simulink model "geometric_control_load"  (R2025a)
settings: Solver=ode15s  StartTime=0.0  StopTime=T_total  FixedStep=0.01  RelTol=1e-9
InitFcn:
  | close all;
  | clear all;
  | %% Parameters
  | mQ = 0.5;
  | mL = 0.1;
  | J = [2.32e-3,0,0;0,2.32e-3,0;0,0,4e-3];
  | g = 9.81;
  | e1 = [1;0;0];
  | e2 = [0;1;0];
  | e3 = [0;0;1];
  | l = 1;
  | type_traj = 0; % 0 elliptical, 1 multi-frequency
  | 
  | %% Initial Condition
  | if type_traj == 0
  |     xL = [0;0.8;1];
  |     vL = zeros(3,1);
  |     th = 125*pi/180;
  |     q = [-sin(th);0;cos(th)];
  |     omega = [0;0;0];
  |     R = [1 0 0;0 1 0;0 0 1];
  |     Omega = [0;0;0];
  | else
  |     xL = [0;1;3];
  |     vL = zeros(3,1);
  |     th = 178*pi/180;
  |     q = [-sin(th);0;-cos(th)];
  |     omega = [0;0;0];
  |     R = [-1 0 0;0 1 0;0 0 -1];
  |     Omega = [0;0;0];
  | end
  | 
  | x_0 = [xL; q; reshape(R, 9,1); vL ;omega; Omega];
  | T_total = 10;
settings Model: Creator=fabioruggiero  LastModifiedBy=maist
settings ModelReferenceCC: EnableRefExpFcnMdlSchedulingChecks=on
settings RTWCC: GPUComputeCapability=3.5

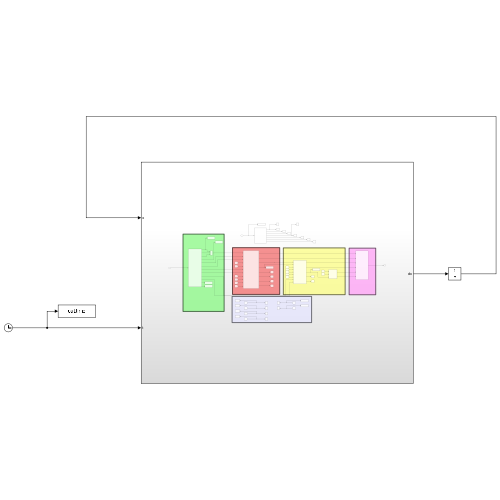
[thumbnail: Simulink's stored preview of the top-level diagram]
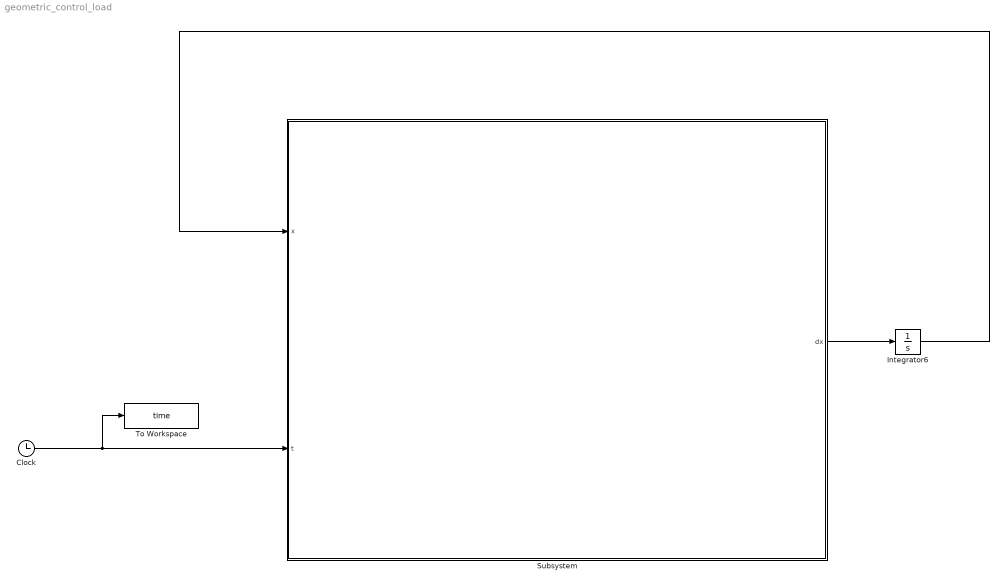
== system geometric_control_load ==
  Clock : Clock
  Integrator6 : Integrator  InitialCondition=x_0
  Subsystem : Subsystem
  To Workspace : ToWorkspace  VariableName=time  SampleTime=-1
      settings: Save2DSignal=2-D array (concatenate along first dimension)
  wires:
  Subsystem/1(dx) -> Integrator6/1
  Integrator6/1 -> Subsystem/1(x)
  Clock/1 -> To Workspace/1, Subsystem/2(t)

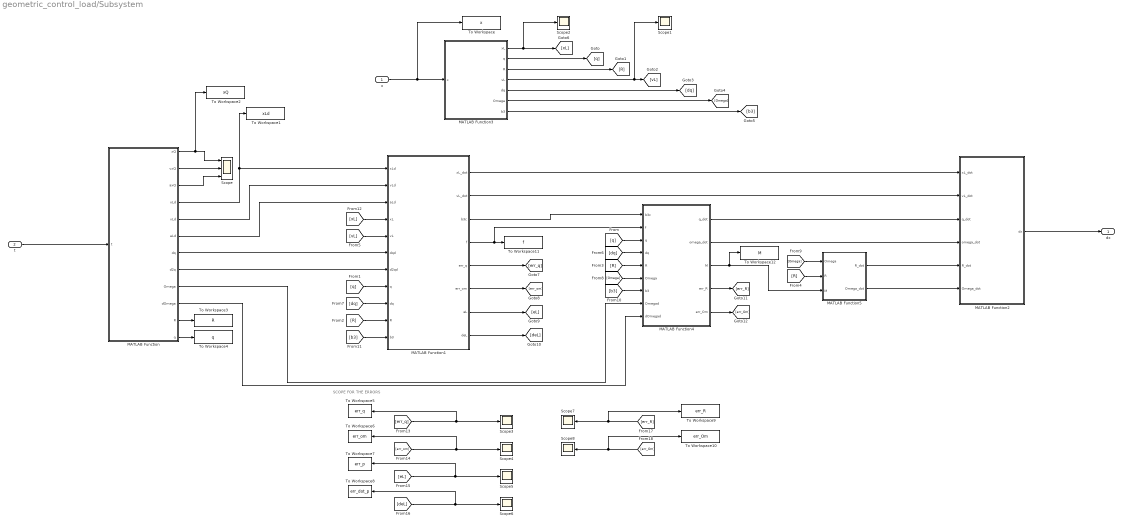
== system geometric_control_load/Subsystem ==
  note: SCOPE FOR THE ERRORS
  x : Inport
  t : Inport  Port=2
  MATLAB Function : MATLAB Function  TreatAsAtomicUnit=on
  MATLAB Function1 : MATLAB Function  TreatAsAtomicUnit=on
  MATLAB Function2 : MATLAB Function  TreatAsAtomicUnit=on
  MATLAB Function3 : MATLAB Function  TreatAsAtomicUnit=on
  MATLAB Function4 : MATLAB Function  TreatAsAtomicUnit=on
  MATLAB Function5 : MATLAB Function  TreatAsAtomicUnit=on
  Scope : Scope  NumInputPorts=3
      settings: ActiveDisplayYMinimum=-2.78929  ActiveDisplayYMaximum=4.74636
  Scope{1..8} (8 alike) : Scope
      Scope1 settings: ActiveDisplayYMinimum=-3.85696  ActiveDisplayYMaximum=4.72111
      Scope2 settings: ActiveDisplayYMinimum=-4.5090813739602247  ActiveDisplayYMaximum=5.0436767590166554
      Scope3 settings: ActiveDisplayYMinimum=-1.0972642217159343  ActiveDisplayYMaximum=1.1831120061993132
      Scope4 settings: ActiveDisplayYMinimum=-1  ActiveDisplayYMaximum=1  DataLoggingVariableName=ScopeData2
      Scope5 settings: ActiveDisplayYMinimum=-6.4063703352333583  ActiveDisplayYMaximum=2.3784855928037065  DataLoggingVariableName=ScopeData3
      Scope6 settings: ActiveDisplayYMinimum=-1  ActiveDisplayYMaximum=1  DataLoggingVariableName=ScopeData4
      Scope7 settings: ActiveDisplayYMinimum=-0.96768549587704089  ActiveDisplayYMaximum=1.1643255351100141  DataLoggingVariableName=ScopeData5
      Scope8 settings: DataLoggingVariableName=ScopeData6
  To Workspace : ToWorkspace  VariableName=x  SampleTime=-1
      settings: Save2DSignal=2-D array (concatenate along first dimension)
  To Workspace1 : ToWorkspace  VariableName=xLd  SampleTime=-1
      settings: Save2DSignal=2-D array (concatenate along first dimension)
  To Workspace10 : ToWorkspace  VariableName=err_Om  SampleTime=-1
      settings: Save2DSignal=2-D array (concatenate along first dimension)
  To Workspace11 : ToWorkspace  VariableName=f  SampleTime=-1
      settings: Save2DSignal=2-D array (concatenate along first dimension)
  To Workspace12 : ToWorkspace  VariableName=M  SampleTime=-1
      settings: Save2DSignal=2-D array (concatenate along first dimension)
  To Workspace2 : ToWorkspace  VariableName=xQ  SampleTime=-1
      settings: Save2DSignal=2-D array (concatenate along first dimension)
  To Workspace3 : ToWorkspace  VariableName=R  SampleTime=-1
  To Workspace4 : ToWorkspace  VariableName=q  SampleTime=-1
      settings: Save2DSignal=2-D array (concatenate along first dimension)
  To Workspace5 : ToWorkspace  VariableName=err_q  SampleTime=-1
      settings: Save2DSignal=2-D array (concatenate along first dimension)
  To Workspace6 : ToWorkspace  VariableName=err_om  SampleTime=-1
      settings: Save2DSignal=2-D array (concatenate along first dimension)
  To Workspace7 : ToWorkspace  VariableName=err_p  SampleTime=-1
      settings: Save2DSignal=2-D array (concatenate along first dimension)
  To Workspace8 : ToWorkspace  VariableName=err_dot_p  SampleTime=-1
      settings: Save2DSignal=2-D array (concatenate along first dimension)
  To Workspace9 : ToWorkspace  VariableName=err_R  SampleTime=-1
      settings: Save2DSignal=2-D array (concatenate along first dimension)
  dx : Outport
  wires:
  MATLAB Function2/1(dx) -> dx/1
  x/1 -> To Workspace/1, MATLAB Function3/1(x)
  MATLAB Function3/5(dq) -> [dq]
  MATLAB Function3/7(b3) -> [b3]
  MATLAB Function/8(d2q) -> MATLAB Function1/7(d2qd)
  MATLAB Function/10(dOmega) -> MATLAB Function4/9(dOmegad)
  MATLAB Function3/1(xL) -> Scope2/1, [xL]
  MATLAB Function3/2(q) -> [q]
  MATLAB Function3/3(R) -> [R]
  MATLAB Function3/6(Omega) -> [Omega]
  MATLAB Function1/3(b3c) -> MATLAB Function4/1(b3c)
  MATLAB Function/9(Omega) -> MATLAB Function4/8(Omegad)
  MATLAB Function1/1(xL_dot) -> MATLAB Function2/1(xL_dot)
  MATLAB Function1/2(vL_dot) -> MATLAB Function2/2(vL_dot)
  MATLAB Function4/1(q_dot) -> MATLAB Function2/3(q_dot)
  MATLAB Function5/1(R_dot) -> MATLAB Function2/5(R_dot)
  MATLAB Function5/2(Omega_dot) -> MATLAB Function2/6(Omega_dot)
  MATLAB Function1/4(f) -> MATLAB Function4/2(f), To Workspace11/1
  MATLAB Function4/3(M) -> MATLAB Function5/3(M), To Workspace12/1
  MATLAB Function/1(xQ) -> To Workspace2/1, Scope/1
  MATLAB Function/4(xLd) -> MATLAB Function1/1(xLd), To Workspace1/1
  MATLAB Function/5(vLd) -> MATLAB Function1/2(vLd)
  MATLAB Function/6(aLd) -> MATLAB Function1/3(aLd)
  MATLAB Function/7(dq) -> MATLAB Function1/6(dqd)
  MATLAB Function1/5(err_q) -> [err_q]
  MATLAB Function1/6(err_om) -> [err_om]
  MATLAB Function1/7(eL) -> [eL]
  MATLAB Function1/8(deL) -> [deL]
  MATLAB Function4/4(err_R) -> [err_R]
  MATLAB Function4/5(err_Om) -> [err_Om]
  MATLAB Function/2(vxQ) -> Scope/2
  MATLAB Function/3(axQ) -> Scope/3
  MATLAB Function/11(R) -> To Workspace3/1
  MATLAB Function/12(q) -> To Workspace4/1
  [q] -> MATLAB Function1/8(q)
  [q] -> MATLAB Function4/3(q)
  [R] -> MATLAB Function1/10(R)
  [R] -> MATLAB Function4/5(R)
  [R] -> MATLAB Function5/2(R)
  [vL] -> MATLAB Function1/5(vL)
  MATLAB Function3/4(vL) -> Scope1/1, [vL]
  [dq] -> MATLAB Function1/9(dq)
  [dq] -> MATLAB Function4/4(dq)
  [Omega] -> MATLAB Function4/6(Omega)
  [Omega] -> MATLAB Function5/1(Omega)
  [b3] -> MATLAB Function1/11(b3)
  [b3] -> MATLAB Function4/7(b3)
  [xL] -> MATLAB Function1/4(xL)
  MATLAB Function4/2(omega_dot) -> MATLAB Function2/4(omega_dot)
  [err_q] -> To Workspace5/1, Scope3/1
  [err_om] -> To Workspace6/1, Scope4/1
  [eL] -> To Workspace7/1, Scope5/1
  [deL] -> To Workspace8/1, Scope6/1
  [err_R] -> To Workspace9/1, Scope7/1
  [err_Om] -> To Workspace10/1, Scope8/1
  t/1 -> MATLAB Function/1(t)

== matlab function geometric_control_load/Subsystem/MATLAB Function1 ==
  data: xLd input; vLd input; aLd input; xL_dot output; vL_dot output; xL input; b3c output; vL input; dqd input; d2qd input; q input; dq input; R input; mQ parameter; f output; b3 input; err_q output; err_om output; eL output; deL output; mL parameter; g parameter; e3 parameter; l parameter
function [xL_dot,vL_dot,b3c,f,err_q,err_om,eL,deL] = Load_Controller(xLd,vLd,aLd,xL,vL,dqd,d2qd,q,dq, R, mQ, b3, mL, g, e3, l)
%% Load Position And Attitude Controller

% Position errors
eL = xL - xLd;
deL = vL - vLd;

epsilon_bar = 0.8;
kp_xy = 0.3/epsilon_bar^2; kd_xy = 0.6/epsilon_bar;
kx = diag([kp_xy kp_xy 2]); kv = diag([kd_xy kd_xy 1.5]);

A = (-kx*eL - kv*deL + (mQ+mL)*(aLd+g*e3) + mQ*l*vec_dot(dq,dq)*q);
qd = -A/norm(A);

epsilon_q = 0.5;
kq = -1.5/epsilon_q^2; kom = -0.8/epsilon_q;
err_q = skew(q)^2*qd;
err_om = dq - cross(cross(qd, dqd), q);

F_pd = -kq*err_q-kom*err_om;
F_ff = (mQ*l)*vec_dot(q, cross(qd,dqd))*cross(q,dq)+...
    (mQ*l)*cross( cross(qd, d2qd), q);
F_n = vec_dot(A,q)*q;

F =  F_pd - F_ff + F_n;

b3c = F/norm(F);

f = vec_dot(F, R(:,3));

%% Load Position Model
xL_dot = vL;
vL_dot = 1/(mQ+mL)*((vec_dot(q,f*b3)-mQ*l*vec_dot(dq,dq))*q-(mQ+mL)*g*e3);

end

 function c = vec_dot(a, b)
        c = a'*b ;
    end
    
    function A = skew(t)
        A = [0 -t(3) t(2) ; t(3) 0 -t(1) ; -t(2) t(1) 0] ;
    end

== matlab function geometric_control_load/Subsystem/MATLAB Function3 ==
  data: x input; xL output; q output; R output; vL output; dq output; Omega output; b3 output
function  [xL,q,R,vL,dq,Omega,b3]=extracting_states(x)
xL = x(1:3);
q = x(4:6);
R = reshape(x(7:15), 3,3);
vL = x(16:18);
omega = x(19:21);
dq = cross(omega, q);

Omega = x(22:24);
b3 = R(:,3);
end

== matlab function geometric_control_load/Subsystem/MATLAB Function4 ==
  data: b3c input; f input; q input; dq input; R input; Omega input; b3 input; Omegad input; dOmegad input; q_dot output; mQ parameter; omega_dot output; M output; err_R output; err_Om output; e1 parameter; J parameter; l parameter
function [q_dot,omega_dot,M,err_R,err_Om] = Quadrotor_Attiitude_Controller(b3c,f,q,dq,R,Omega,b3,Omegad,dOmegad, mQ, e1, J, l)

%% Load Attitude Model
q_dot = dq;
omega_dot = 1/(mQ*l) * cross(-q, f*b3);

%% Quadrotor Attitude Controller
b1d = e1;
b1c = -cross(b3c,cross(b3c,b1d))/norm(cross(b3c,b1d));
Rc = [b1c, cross(b3c,b1c),b3c];
Rd = Rc;

kR = 4 ; kOm = 4 ;
epsilon = 0.1 ; 

err_R = 1/2 * vee_map(Rd'*R - R'*Rd);
err_Om = Omega - R'*Rd*Omegad;
M = -kR/epsilon^2*err_R - kOm/epsilon*err_Om + cross(Omega, J*Omega)...
    - J*(skew(Omega)*R'*Rd*Omegad - R'*Rd*dOmegad);

end
    
    function A = skew(t)
        A = [0 -t(3) t(2) ; t(3) 0 -t(1) ; -t(2) t(1) 0] ;
    end
    
    function t = vee_map(A, force)
        if(nargin == 1)
            force = false ;
        end
        if(~force)
            if(double(sum(abs(diag(A)))) > 1e-2)
                % disp('Error in vee_map() - Nonzero diagonal') ; % Commentato
            end
        end
        t = [A(3,2) ; A(1,3) ; A(2,1)] ;
    end

== matlab function geometric_control_load/Subsystem/MATLAB Function ==
  data: xQ output; vxQ output; axQ output; xLd output; vLd output; aLd output; dq output; d2q output; Omega output; mQ parameter; dOmega output; R output; q output; mL parameter; e1 parameter; g parameter; e3 parameter; l parameter; t input; type_traj parameter
function [xQ,vxQ,axQ,xLd,vLd,aLd,dq,d2q,Omega,dOmega,R,q]...
          = Planner(mQ, mL, e1, g, e3, l, t, type_traj)

%% Trajectories

if type_traj == 0

    % Ellictical Trajectory

    T0 = 2*pi;
    w = 2*pi/T0;% angular velocity
    
    Ax = 0.5;
    Ay = 0.8;
    Az = 1;
    
    
    % Derivative of Load Position
    xLd = [Ax*sin(w*t); Ay*cos(w*t); Az];
    vLd = [Ax*w*cos(w*t);  Ay*-w*sin(w*t); 0];
    aLd = [Ax*-w^2*sin(w*t);  Ay*-w^2*cos(w*t); 0];
    daLd = [Ax*-w^3*cos(w*t);  Ay*w^3*sin(w*t); 0];
    d2aLd = [Ax*w^4*sin(w*t); Ay*w^4*cos(w*t); 0];
    d3aLd = [Ax*w^5*cos(w*t);  Ay*-w^5*sin(w*t); 0];
    d4aLd = [Ax*-w^6*sin(w*t); Ay*w^6*cos(w*t); 0];
else 

    % Sinusoidal Trajectory
    f1 = 1/4;
    f2 = 1/5;
    f3 = 1/7;
    
    a_x = 2;
    a_y = 2.5;
    a_z = 1.5;
    
    % Derivative of Load Position
    xLd = [a_x*(1 - cos(2*pi*f1*t));
        a_y * sin(2*pi*f2*t);
        a_z * cos(2*pi*f3*t)];
    vLd = 2*pi*[f1*a_x*sin(2*pi*f1*t);
        f2*a_y * cos(2*pi*f2*t);
        f3*1.5 * -sin(2*pi*f3*t)];
    aLd = (2*pi)^2*[f1^2*a_x*cos(2*pi*f1*t);
        f2^2*a_y * -sin(2*pi*f2*t);
        f3^2*a_z * -cos(2*pi*f3*t)];
    daLd = (2*pi)^3*[f1^3*a_x*-sin(2*pi*f1*t);
        f2^3*a_y * -cos(2*pi*f2*t);
        f3^3*a_z * sin(2*pi*f3*t)];
    d2aLd = (2*pi)^4*[f1^4*a_x*-cos(2*pi*f1*t);
        f2^4*a_y * sin(2*pi*f2*t);
        f3^4*a_z * cos(2*pi*f3*t)];
    d3aLd = (2*pi)^5*[f1^5*a_x*sin(2*pi*f1*t);
        f2^5*a_y * cos(2*pi*f2*t);
        f3^5*a_z * -sin(2*pi*f3*t)];
    d4aLd = (2*pi)^6*[f1^6*a_x*cos(2*pi*f1*t);
        f2^6*a_y * -sin(2*pi*f2*t);
        f3^6*a_z * -cos(2*pi*f3*t)];
end

% Tension Cable and Directional Vector

Tq = -mL*(aLd + g*e3) ;
norm_Tq = norm(Tq);
q = Tq / norm_Tq;
xQ = xLd - l*q;

dTq = -mL*daLd ;
dnorm_Tq = 1/norm_Tq * vec_dot(Tq, dTq) ;
dq = (dTq - q*dnorm_Tq) / norm_Tq ;


d2Tq = -mL*d2aLd ;
d2norm_Tq = ( vec_dot(dTq, dTq) + vec_dot(Tq, d2Tq) - dnorm_Tq^2 ) / norm_Tq ;
d2q = ( d2Tq - dq*dnorm_Tq - q*d2norm_Tq - dq*dnorm_Tq) / norm_Tq ;

d3Tq = -mL*d3aLd ;
d3norm_Tq = ( 2*vec_dot(d2Tq, dTq) + vec_dot(dTq, d2Tq)+vec_dot(Tq, d3Tq) - 3*dnorm_Tq*d2norm_Tq) / norm_Tq ;
d3q = (d3Tq - d2q*dnorm_Tq-dq*d2norm_Tq - dq*d2norm_Tq-q*d3norm_Tq - d2q*dnorm_Tq-dq*d2norm_Tq - d2q*dnorm_Tq) / norm_Tq ;

d4Tq = -mL*d4aLd;
d4norm_Tq = ( 2*vec_dot(d3Tq, dTq)+2*vec_dot(d2Tq, d2Tq) + vec_dot(d2Tq, d2Tq)+vec_dot(dTq, d3Tq) + vec_dot(dTq, d3Tq)+vec_dot(Tq, d4Tq) - 3*d2norm_Tq^2-3*dnorm_Tq*d3norm_Tq ...
    - d3norm_Tq*dnorm_Tq) / norm_Tq ;
d4q = ( d4Tq - d3q*dnorm_Tq-d2q*d2norm_Tq - d2q*d2norm_Tq-dq*d3norm_Tq - d2q*d2norm_Tq-dq*d3norm_Tq - dq*d3norm_Tq-q*d4norm_Tq ...
    - d3q*dnorm_Tq-d2q*d2norm_Tq - d2q*d2norm_Tq-dq*d3norm_Tq - d3q*dnorm_Tq-d2q*d2norm_Tq - d3q*dnorm_Tq ) / norm_Tq ;

% Derivatives of Quadrotor's Position
vxQ = vLd - l*dq;
axQ = aLd - l*d2q;
daxQ = daLd - l*d3q;
d2axQ = d2aLd - l*d4q;

b1d = e1;
db1d = zeros(3,1);
d2b1d = zeros(3,1);

fb3 = mQ*(axQ+g*e3) - Tq;
norm_fb3 = norm(fb3);
b3 = fb3 / norm_fb3;
b3_b1d = cross(b3, b1d);
norm_b3_b1d = norm(b3_b1d);
b1 = - cross(b3, b3_b1d) / norm_b3_b1d;
b2 = cross(b3, b1);
R = [b1 b2 b3];

dfb3 = mQ*(daxQ) - dTq;
dnorm_fb3 = vec_dot(fb3, dfb3) / norm_fb3;
db3 = (dfb3*norm_fb3 - fb3*dnorm_fb3) / norm_fb3^2;
db3_b1d = cross(db3, b1d) + cross(b3, db1d);
dnorm_b3_b1d = vec_dot(b3_b1d, db3_b1d) / norm_b3_b1d;
db1 = (-cross(db3,b3_b1d)-cross(b3,db3_b1d) - b1*dnorm_b3_b1d) / norm_b3_b1d;
db2 = cross(db3, b1) + cross(b3, db1);
dR = [db1 db2 db3];
Omega = vee_map(R'*dR);

d2fb3 = mQ*(d2axQ) - d2Tq ;
d2norm_fb3 = (vec_dot(dfb3, dfb3)+vec_dot(fb3, d2fb3) - dnorm_fb3*dnorm_fb3) / norm_fb3 ;
d2b3 = ( (d2fb3*norm_fb3+dfb3*dnorm_fb3 - dfb3*dnorm_fb3-fb3*d2norm_fb3)*norm_fb3^2 - db3*norm_fb3^2*2*norm_fb3*dnorm_fb3 ) / norm_fb3^4 ;
d2b3_b1d = cross(d2b3, b1d)+cross(db3, db1d) + cross(db3, db1d)+cross(b3, d2b1d) ;
d2norm_b3_b1d = ( (vec_dot(db3_b1d,db3_b1d)+vec_dot(b3_b1d,d2b3_b1d))*norm_b3_b1d - vec_dot(b3_b1d, db3_b1d)*dnorm_b3_b1d ) / norm_b3_b1d^2 ;
d2b1 = ( (-cross(d2b3,b3_b1d)-cross(db3,db3_b1d) - cross(db3,db3_b1d)-cross(b3,d2b3_b1d) - db1*dnorm_b3_b1d-b1*d2norm_b3_b1d )*norm_b3_b1d - db1*norm_b3_b1d*dnorm_b3_b1d ) / norm_b3_b1d^2 ;
d2b2 = cross(d2b3, b1)+cross(db3, db1) + cross(db3, db1)+cross(b3, d2b1) ;
d2R = [d2b1 d2b2 d2b3] ;
dOmega = vee_map( dR'*dR + R'*d2R ) ; 

end
    function c = vec_dot(a, b)
        c = a'*b ;
    end
    
    function t = vee_map(A, force)
        if(nargin == 1)
            force = false ;
        end
        if(~force)
            if(double(sum(abs(diag(A)))) > 1e-2)
                % disp('Error in vee_map() - Nonzero diagonal') ;
            end
        end
        t = [A(3,2) ; A(1,3) ; A(2,1)] ;
    end

== matlab function geometric_control_load/Subsystem/MATLAB Function5 ==
  data: Omega input; R_dot output; R input; M input; Omega_dot output; J parameter
function [R_dot,Omega_dot] = Quadrotor_Attitude(Omega,R,M,J)

%% Quadrotor Attitude Model
R_dot = R*skew(Omega);
Omega_dot = inv(J)*( -cross(Omega, J*Omega) + M );
end

function A = skew(t)
        A = [0 -t(3) t(2) ; t(3) 0 -t(1) ; -t(2) t(1) 0] ;
    end

== matlab function geometric_control_load/Subsystem/MATLAB Function2 ==
  data: xL_dot input; vL_dot input; dx output; q_dot input; omega_dot input; R_dot input; Omega_dot input
function dx = output(xL_dot,vL_dot,q_dot,omega_dot,R_dot,  Omega_dot)
dx = [xL_dot; q_dot; reshape(R_dot, 9,1); vL_dot; omega_dot; Omega_dot];
end
